simulink model "model2"  (R2021b)
settings: Solver=VariableStepAuto  StartTime=0.0  StopTime=10.0  RelTol=1e-3
undefined symbols (not defined in the file): c1, c2, k1, k2, m1, m2
settings Model: Creator=szczy  LastModifiedBy=szczy

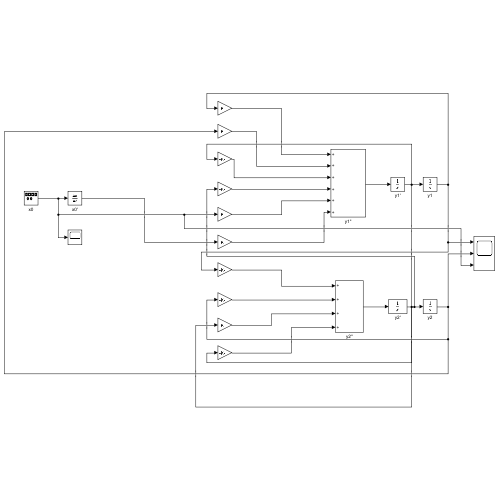
[thumbnail: Simulink's stored preview of the top-level diagram]
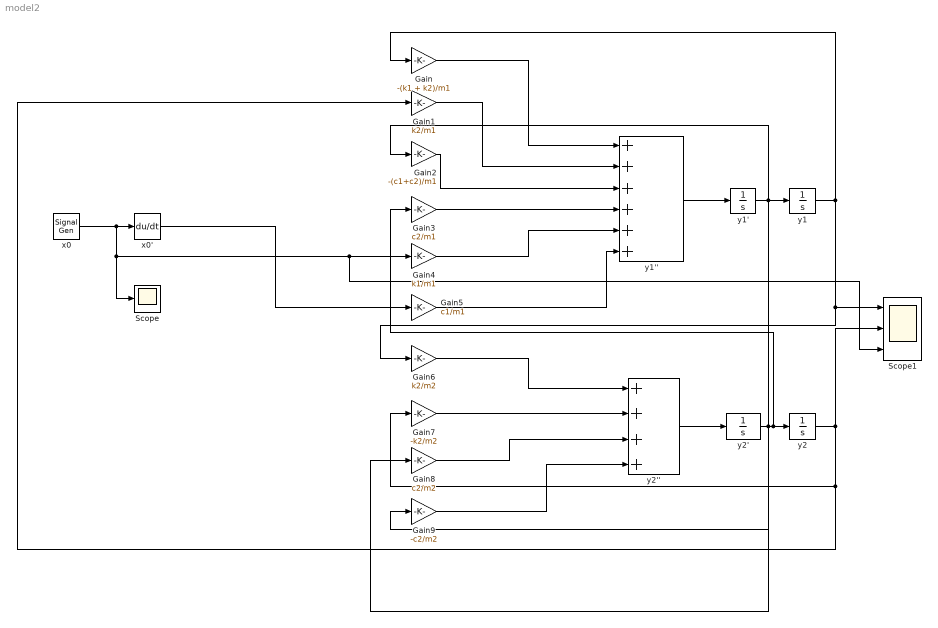
== system model2 ==
  Gain : Gain  Gain=-(k1 + k2)/m1
  Gain1 : Gain  Gain=k2/m1
  Gain2 : Gain  Gain=-(c1+c2)/m1
  Gain3 : Gain  Gain=c2/m1
  Gain4 : Gain  Gain=k1/m1
  Gain5 : Gain  Gain=c1/m1
  Gain6 : Gain  Gain=k2/m2
  Gain7 : Gain  Gain=-k2/m2
  Gain8 : Gain  Gain=c2/m2
  Gain9 : Gain  Gain=-c2/m2
  Scope : Scope
  Scope1 : Scope  NumInputPorts=3
  x0 : SignalGenerator  WaveForm=square  Units=rad/sec
  x0' : Derivative
  y1 : Integrator
  y1' : Integrator
  y1'' : Sum  Inputs=++++++
  y2 : Integrator
  y2' : Integrator
  y2'' : Sum  Inputs=++++
  wires:
  x0/1 -> Scope1/3, Gain4/1, Scope/1, x0'/1
  Gain/1 -> y1''/1
  Gain1/1 -> y1''/2
  Gain2/1 -> y1''/3
  Gain3/1 -> y1''/4
  Gain4/1 -> y1''/5
  Gain5/1 -> y1''/6
  Gain6/1 -> y2''/1
  Gain7/1 -> y2''/2
  Gain8/1 -> y2''/3
  Gain9/1 -> y2''/4
  y1''/1 -> y1'/1
  y1'/1 -> Gain2/1, Gain8/1, y1/1
  y1/1 -> Gain6/1, Scope1/1, Gain/1
  y2''/1 -> y2'/1
  y2'/1 -> Gain9/1, Gain3/1, y2/1
  y2/1 -> Scope1/2, Gain7/1, Gain1/1
  x0'/1 -> Gain5/1
